simulink subsystem "OptPath_Gen"  (R2024a)
settings: Solver=VariableStepAuto  StartTime=0.0  StopTime=10.0  RelTol=1e-3
settings Model: Creator=User  LastModifiedBy=User

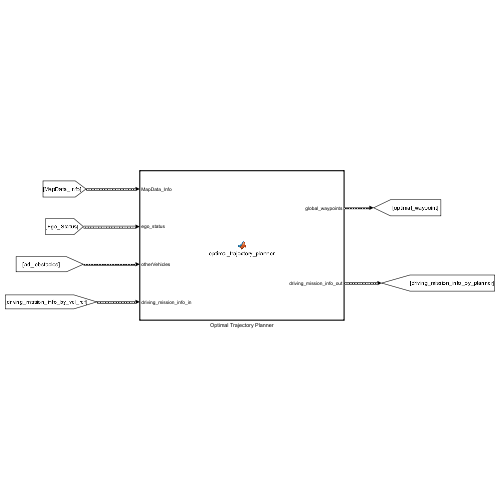
[thumbnail: Simulink's stored preview of the top-level diagram]
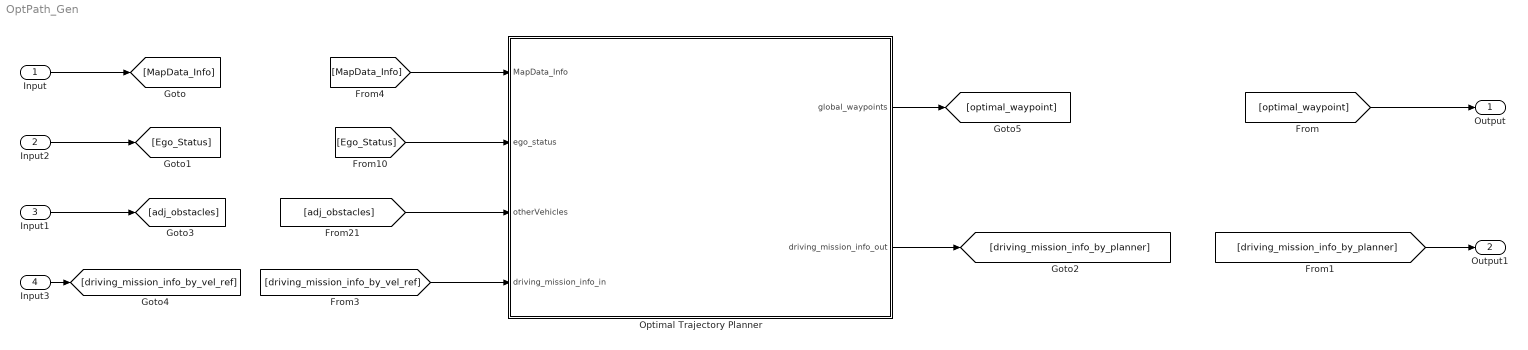
== system OptPath_Gen ==
  Input : Inport
  Input2 : Inport  Port=2
  Input1 : Inport  Port=3
  Input3 : Inport  Port=4
  Optimal Trajectory Planner : MATLAB Function  TreatAsAtomicUnit=on
  Output : Outport
  Output1 : Outport  Port=2
  wires:
  Optimal Trajectory Planner/2(driving_mission_info_out) -> [driving_mission_info_by_planner]
  [driving_mission_info_by_vel_ref] -> Optimal Trajectory Planner/4(driving_mission_info_in)
  [MapData_Info] -> Optimal Trajectory Planner/1(MapData_Info)
  [Ego_Status] -> Optimal Trajectory Planner/2(ego_status)
  [adj_obstacles] -> Optimal Trajectory Planner/3(otherVehicles)
  Optimal Trajectory Planner/1(global_waypoints) -> [optimal_waypoint]
  Input/1 -> [MapData_Info]
  Input2/1 -> [Ego_Status]
  Input1/1 -> [adj_obstacles]
  Input3/1 -> [driving_mission_info_by_vel_ref]
  [optimal_waypoint] -> Output/1
  [driving_mission_info_by_planner] -> Output1/1

== matlab function OptPath_Gen/Optimal Trajectory Planner ==
  settings: sampleTime=0.05
  data: MapData_Info input; ego_status input; global_waypoints output size=[50 2]; otherVehicles input; driving_mission_info_in input Bus: busDrivingMissionInfo; driving_mission_info_out output Bus: busDrivingMissionInfo
function [global_waypoints, driving_mission_info_out]  = optimal_trajectory_planner(MapData_Info, ego_status, otherVehicles, driving_mission_info_in)
    % centerLine: [X, Y]
    % egoState: [x, y, yaw, v, a]
    % otherVehicles: [X, Y, Vx, Vy, Ax, Ay, Yaw, Yawrate]
    % N_pts: 출력할 trajectory 점 개수
    % 출력: x_traj, y_traj - N_pts x 1 trajectory
    %git test
  [global_waypoints, driving_mission_info_out]  = optimal_trajectory_planner_m(MapData_Info, ego_status, otherVehicles, driving_mission_info_in);
end
